simulink model "GS_model"  (R2018b)
settings: Solver=ode5  StartTime=0.0  StopTime=SimuStopTime  FixedStep=T_Simu  RelTol=1e-3
InitFcn:
  | Initial
undefined symbols (not defined in the file or in its folder): Aba10, Aba20, aeroCIP2006_S, aeroCIP2006_X, aeroCIP2006_Y, Agl0, Ass_kS, Ass_n1, Ass_n2, Ass_n3, Ass_n4, Ass_Noise, Ass_R, Ass_Resolution, Ass_TmOrder, AssA_Fix_Abs, AssB_Fix_Abs, AssC_Fix_Abs, AssD_Fix_Abs, AssE_Fix_Aps, AssF_Fix_Aps, C, c_max, c_min, Cd, CenterOfFigNX, CenterOfFigNY, CenterOfFigNZ, CenterOfFigP1, CenterOfFigP2, CenterOfFigPX, CenterOfFigPY, CenterOfFigPZ, Cmu, Crou, DEG2RAD, DiscIntNeverNeededParam, Eg_Dir, Eg_F, Eg_PrepareTime, Eg_r_L_L, Fw_Abf, Fw_Hmax, Fw_J, Fw_Spd0, Fw_Tmax, git_hash_BaseLine, git_hash_Project, Gnss_Noise_Pos, Gnss_Noise_Vel, Gnss_PropgationTime, GyroA_Fix_Abg, GyroA_Noise, GyroB_Fix_Abg, GyroB_Noise, GyroC_Fix_Abg, GyroC_Noise, GyroD_Fix_Abg, GyroD_Noise, h ... (+94)
libraries: simulink x308, sharedutil x46, aerolibutil x37, sharedtransform x31, vrlib x14, aerolibgravity2 x2
(part 1 of 20)
settings Model: PauseTimes=110  ExtModeArmWhenConnect=off  Creator=Think  LastModifiedBy=xiahesong
settings DataIOCC: LimitDataPoints=on  SaveFormat=Array  SaveOutput=off  SaveTime=off  SignalLoggingName=sigsOut
settings DebuggingCC: ReadBeforeWriteMsg=DisableAll  WriteAfterWriteMsg=DisableAll  WriteAfterReadMsg=DisableAll  SaveWithParameterizedLinksMsg=none  MergeDetectMultiDrivingBlocksExec=none  SignalResolutionControl=None  InheritedTsInSrcMsg=none  MultiTaskDSMMsg=none  IntegerOverflowMsg=none  ParameterPrecisionLossMsg=none  ParameterTunabilityLossMsg=none  RootOutportRequireBusObject=error  AllowSymbolicDim=off  StrictBusMsg=ErrorOnBusTreatedAsVector  SFUnexpectedBacktrackingDiag=warning  SFNoUnconditionalDefaultTransitionDiag=warning  IntegerSaturationMsg=none
settings HardwareCC: ProdBitPerPointer=32  ProdBitPerSizeT=32  ProdBitPerPtrDiffT=32  ProdLargestAtomicFloat=None  ProdWordSize=32  ProdHWDeviceType=Intel->x86/Pentium
settings ModelReferenceCC: UpdateModelReferenceTargets=IfOutOfDate  PropagateSignalLabelsOutOfModel=off
settings SFSimCC: SFSimEcho=off  SimUseLocalCustomCode=off
settings RTWCC: SystemTargetFile=NIVeriStand.tlc  TemplateMakefile=NIVeriStand_vc.tmf  Description=DEPRECATED: NI VeriStand Pharlap Real-Time Targets (MATLAB R2018b or earlier)  RTWUseLocalCustomCode=off  RTWCompilerOptimization=on
settings CodeAppCC: StateflowObjectComments=on
settings STFCustomTargetCC: MatFileLogging=on  GRTInterface=on  SystemTargetFile=NIVeriStand.tlc
settings GRTTargetCC: TargetLangStandard=C89/C90 (ANSI)  ParMdlRefBuildCompliant=off  CompOptLevelCompliant=off  ConcurrentExecutionCompliant=off  CombineOutputUpdateFcns=off  CPPClassGenCompliant=off  GRTInterface=on  UseToolchainInfoCompliant=off
settings ConfigComp: CovMetricSettings=dw  CovHtmlReporting=on  CovSaveCumulativeToWorkspaceVar=on  CovSaveSingleToWorkspaceVar=on  CovExternalEMLEnable=off  CovSFcnEnable=off

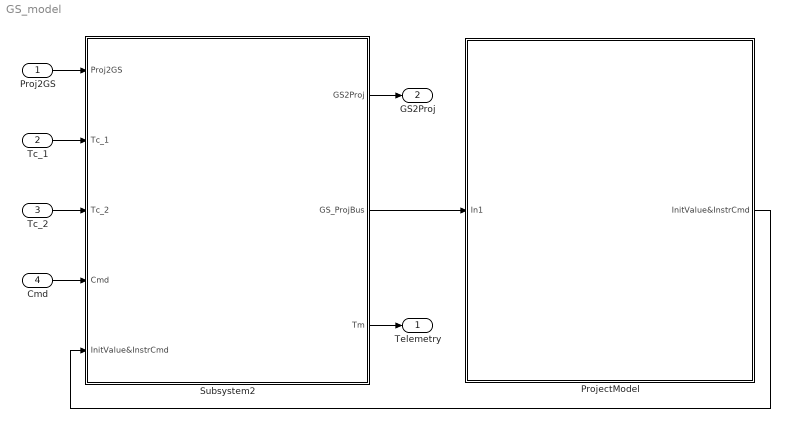
== system GS_model ==
  Proj2GS : Inport
  Tc_1 : Inport  Port=2
  Tc_2 : Inport  Port=3
  Cmd : Inport  Port=4
  ProjectModel : Subsystem
      mask Display: disp('Project Model')
  Subsystem2 : Subsystem
      mask Display: disp('GS_model');
  Telemetry : Outport
  GS2Proj : Outport  Port=2  PortDimensions=166
  wires:
  Tc_1/1 -> Subsystem2/2(Tc_1)
  Tc_2/1 -> Subsystem2/3(Tc_2)
  Cmd/1 -> Subsystem2/4(Cmd)
  Subsystem2/3(Tm) -> Telemetry/1
  Proj2GS/1 -> Subsystem2/1(Proj2GS)
  Subsystem2/1(GS2Proj) -> GS2Proj/1
  ProjectModel/1(InitValue&InstrCmd) -> Subsystem2/5(InitValue&InstrCmd)
  Subsystem2/2(GS_ProjBus) -> ProjectModel/1(In1)

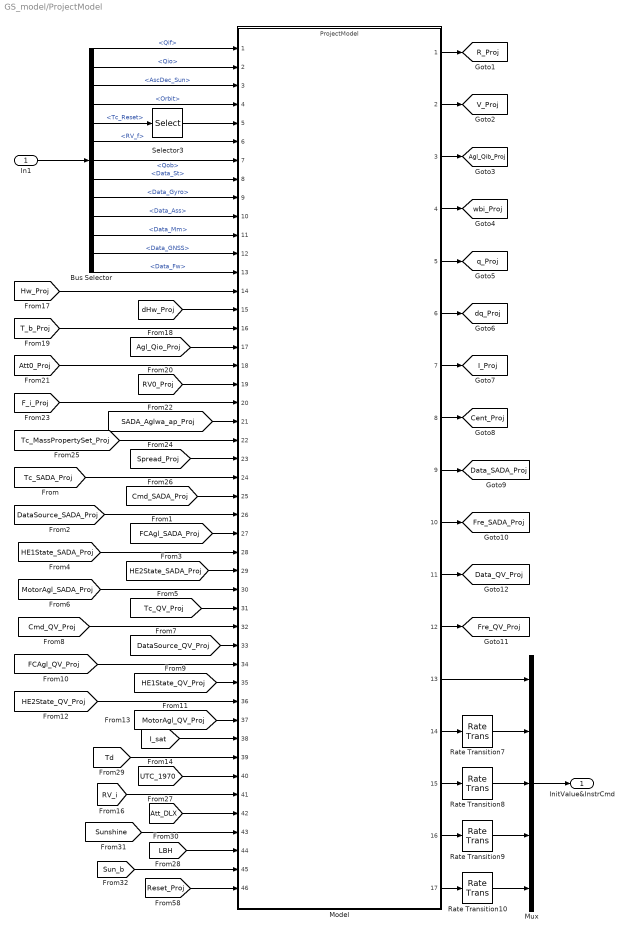
== system GS_model/ProjectModel ==
  In1 : Inport
  Bus Selector : BusSelector  OutputSignals=Qif,Qio,AscDec_Sun,Orbit,Tc_Reset,RV_f,Qob,Data_St,Data_Gyro,Data_Ass,Data_Mm,Data_GNSS,Data_Fw
  Model : ModelReference  ModelNameDialog=ProjectModel  SimulationMode=Normal  ModelReferenceVersion=1.5009
  Mux : Mux  Inputs=5
  Rate Transition{7..10} (4 alike) : RateTransition  OutPortSampleTime=T_Simu
  Selector3 : Selector  InputPortWidth=2  IndexOptions=Index vector (dialog)  Indices=2  OutputSizes=1
  InitValue&InstrCmd : Outport
  tag scope: Agl_Qib_Proj=global, Cent_Proj=global, Data_QV_Proj=global, Data_SADA_Proj=global, Fre_QV_Proj=global, Fre_SADA_Proj=global, I_Proj=global, R_Proj=global, V_Proj=global, dq_Proj=global, q_Proj=global, wbi_Proj=global
  wires:
  Rate Transition8/1 -> Mux/3
  Rate Transition10/1 -> Mux/5
  Rate Transition7/1 -> Mux/2
  Rate Transition9/1 -> Mux/4
  Mux/1 -> InitValue&InstrCmd/1
  Model/1 -> [R_Proj]
  Model/2 -> [V_Proj]
  Model/3 -> [Agl_Qib_Proj]
  Model/4 -> [wbi_Proj]
  Model/5 -> [q_Proj]
  Model/6 -> [dq_Proj]
  Model/7 -> [I_Proj]
  Model/8 -> [Cent_Proj]
  Model/9 -> [Data_SADA_Proj]
  Model/10 -> [Fre_SADA_Proj]
  Model/11 -> [Data_QV_Proj]
  Model/12 -> [Fre_QV_Proj]
  Model/15 -> Rate Transition8/1
  Model/14 -> Rate Transition7/1
  Model/17 -> Rate Transition10/1
  Model/16 -> Rate Transition9/1
  Model/13 -> Mux/1
  In1/1 -> Bus Selector/1
  [HE1State_QV_Proj] -> Model/35
  [MotorAgl_QV_Proj] -> Model/37
  [SADA_Aglwa_ap_Proj] -> Model/21
  [FCAgl_QV_Proj] -> Model/34
  [DataSource_QV_Proj] -> Model/33
  [MotorAgl_SADA_Proj] -> Model/30
  [Tc_QV_Proj] -> Model/31
  [T_b_Proj] -> Model/16
  [FCAgl_SADA_Proj] -> Model/27
  [Spread_Proj] -> Model/23
  [Cmd_SADA_Proj] -> Model/25
  [HE2State_QV_Proj] -> Model/36
  [Agl_Qio_Proj] -> Model/17
  [Tc_SADA_Proj] -> Model/24
  [RV_i] -> Model/41
  [F_i_Proj] -> Model/20
  [Cmd_QV_Proj] -> Model/32
  [dHw_Proj] -> Model/15
  [UTC_1970] -> Model/40
  [HE1State_SADA_Proj] -> Model/28
  [I_sat] -> Model/38
  [HE2State_SADA_Proj] -> Model/29
  [Att0_Proj] -> Model/18
  [RV0_Proj] -> Model/19
  [DataSource_SADA_Proj] -> Model/26
  [Tc_MassPropertySet_Proj] -> Model/22
  [Td] -> Model/39
  [Hw_Proj] -> Model/14
  [Sunshine] -> Model/43
  [Att_DLX] -> Model/42
  [LBH] -> Model/44
  [Sun_b] -> Model/45
  [Reset_Proj] -> Model/46
  Bus Selector/1 -> Model/1  "<Qif>"
  Bus Selector/2 -> Model/2  "<Qio>"
  Bus Selector/3 -> Model/3  "<AscDec_Sun>"
  Bus Selector/4 -> Model/4  "<Orbit>"
  Bus Selector/5 -> Selector3/1  "<Tc_Reset>"
  Bus Selector/6 -> Model/6  "<RV_f>"
  Bus Selector/7 -> Model/7  "<Qob>"
  Bus Selector/8 -> Model/8  "<Data_St>"
  Bus Selector/9 -> Model/9  "<Data_Gyro>"
  Bus Selector/10 -> Model/10  "<Data_Ass>"
  Bus Selector/11 -> Model/11  "<Data_Mm>"
  Bus Selector/12 -> Model/12  "<Data_GNSS>"
  Bus Selector/13 -> Model/13  "<Data_Fw>"
  Selector3/1 -> Model/5

== system GS_model/Subsystem2 ==
  Proj2GS : Inport
  Tc_1 : Inport  Port=2
  Tc_2 : Inport  Port=3
  Cmd : Inport  Port=4
  InitValue&InstrCmd : Inport  Port=5
  " " : Subsystem
      mask Display: disp('Telemetry')
  Bus Creator : BusCreator  Inputs=13
  EquipmentCmd : Subsystem
      mask Display: disp(['Instrument','\n','\n','Cmd'])
  Subsystem : Subsystem
      mask Display: disp('AOCS Model')
  Subsystem1 : Subsystem
      mask Display: disp('Mapping')
  Tc : Subsystem
      mask Display: disp('TC')
  GS2Proj : Outport  PortDimensions=166
  GS_ProjBus : Outport  Port=2
  Tm : Outport  Port=3
  wires:
  InitValue&InstrCmd/1 -> EquipmentCmd/3(InitValue&InstrCmd), Tc/3(InitValue&InstrCmd)
  Tc_2/1 -> Tc/2(Tc_2)
  Cmd/1 -> EquipmentCmd/2(Cmd)
  Tc_1/1 -> Tc/1(Tc_1)
  " "/1(Tm) -> Tm/1
  Tc/18(Tc_Fw) -> Subsystem/18(Tc_Fw), EquipmentCmd/1(Tc_Fw)
  Proj2GS/1 -> Subsystem1/1(In1)
  Subsystem1/1(Out1) -> GS2Proj/1
  Tc/1(Tc_MassProperty) -> Subsystem/1(Tc_MassPropertySet)
  Tc/2(Tc_Sunshine) -> Subsystem/2(Tc_Sunshine)
  Tc/3(Tc_Reset) -> Subsystem/3(Reset)
  Tc/4(Tc_Time0) -> Subsystem/4(Tc_Time0)
  Tc/5(Tc_Orbit0) -> Subsystem/5(Tc_Orbit0)
  Tc/6(Tc_Att0) -> Subsystem/6(Tc_Att0)
  Tc/7(Tc_RemanMag) -> Subsystem/7(Tc_RemanMag)
  Tc/8(Tc_TdCoff) -> Subsystem/8(Tc_TdCoff)
  Tc/9(Tc_St) -> Subsystem/9(Tc_St)
  Tc/10(Tc_Gyro) -> Subsystem/10(Tc_Gyro)
  Tc/11(Tc_Ass) -> Subsystem/11(Tc_Ass)
  Tc/12(Tc_Mm) -> Subsystem/12(Tc_Mm)
  Tc/13(Tc_GNSS) -> Subsystem/13(Tc_GNSS)
  Tc/14(Tc_Mt) -> Subsystem/14(Tc_Mt)
  Tc/15(Tc_SADA) -> Subsystem/15(Tc_SADA)
  Tc/16(Tc_QV) -> Subsystem/16(Tc_QV)
  Tc/17(Tc_Engine) -> Subsystem/17(Tc_Engine)
  Tc/19(Tc_Spread0) -> Subsystem/19(Tc_Spread0)
  EquipmentCmd/1(Cmd_Spread) -> Subsystem/20(Cmd_Spread)
  EquipmentCmd/2(Cmd_Fw) -> Subsystem/21(Cmd_Fw)
  EquipmentCmd/3(Cmd_Mt) -> Subsystem/22(Cmd_Mt)
  EquipmentCmd/4(Cmd_Motor) -> Subsystem/23(Cmd_Motor)
  EquipmentCmd/5(Cmd_Engine) -> Subsystem/24(Cmd_Engine)
  Subsystem/1(Qif) -> Bus Creator/1  "Qif"
  Subsystem/2(Qio) -> Bus Creator/2  "Qio"
  Subsystem/14(Data_St1) -> " "/1(Data_St)
  Subsystem/15(Data_Gyro1) -> " "/2(Data_Gyro)
  Subsystem/16(Data_Ass1) -> " "/3(Data_Ass)
  Subsystem/17(Data_Mm1) -> " "/4(Data_Mm)
  Subsystem/18(Data_GNSS1) -> " "/5(Data_GNSS)
  Subsystem/19(Data_Fw1) -> " "/6(Data_Fw)
  Subsystem/20(Data_Mt) -> " "/7(Data_Mt)
  Subsystem/21(Data_SADA) -> " "/8(Data_SADA)
  Subsystem/22(Data_QV) -> " "/9(Data_QV)
  Subsystem/3(AscDec_Sun) -> Bus Creator/3  "AscDec_Sun"
  Subsystem/4(Orbit) -> Bus Creator/4  "Orbit"
  Subsystem/5(Tc_Reset) -> Bus Creator/5  "Tc_Reset"
  Subsystem/6(RV_f) -> Bus Creator/6  "RV_f"
  Subsystem/7(Qob) -> Bus Creator/7  "Qob"
  Subsystem/8(Data_St) -> Bus Creator/8  "Data_St"
  Subsystem/9(Data_Gyro) -> Bus Creator/9  "Data_Gyro"
  Subsystem/10(Data_Ass) -> Bus Creator/10  "Data_Ass"
  Subsystem/11(Data_Mm) -> Bus Creator/11  "Data_Mm"
  Subsystem/12(Data_GNSS) -> Bus Creator/12  "Data_GNSS"
  Subsystem/13(Data_Fw) -> Bus Creator/13  "Data_Fw"
  Bus Creator/1 -> GS_ProjBus/1

== system GS_model/Subsystem2/  ==
  Data_St : Inport
  Data_Gyro : Inport  Port=2
  Data_Ass : Inport  Port=3
  Data_Mm : Inport  Port=4
  Data_GNSS : Inport  Port=5
  Data_Fw : Inport  Port=6
  Data_Mt : Inport  Port=7
  Data_SADA : Inport  Port=8
  Data_QV : Inport  Port=9
  DynTelemetry : Subsystem
      mask Display: disp('TM_Dyn')
  Hash : Subsystem
      mask Display: disp('TM_Hash')
  Mux : Mux  Inputs=11
  Reshape : Reshape  OutputDimensionality=Row vector (2-D)
  Subsystem : Subsystem
      mask Display: disp('TM_Ass');
  Subsystem1 : Subsystem
      mask Display: disp('TM_SADA');
  Subsystem2 : Subsystem
      mask Display: disp('TM_QV');
  Tm : Outport  VectorParamsAs1DForOutWhenUnconnected=on
  wires:
  DynTelemetry/1(DynTelemetry) -> Mux/1
  Hash/1(Out1) -> Mux/2
  Data_St/1 -> Mux/3
  Data_Gyro/1 -> Mux/4
  Data_Mm/1 -> Mux/5
  Data_GNSS/1 -> Mux/7
  Data_Fw/1 -> Mux/8
  Data_Mt/1 -> Mux/9
  Data_SADA/1 -> Subsystem1/1(Data_SADA)
  Data_QV/1 -> Subsystem2/1(Data_QV)
  Mux/1 -> Reshape/1
  Data_Ass/1 -> Subsystem/1(Data_Ass)
  Subsystem/1(Out6) -> Mux/6
  Reshape/1 -> Tm/1
  Subsystem1/1(Out6) -> Mux/10
  Subsystem2/1(Out6) -> Mux/11

== system GS_model/Subsystem2/EquipmentCmd ==
  Tc_Fw : Inport
  Cmd : Inport  Port=2
  InitValue&InstrCmd : Inport  Port=3
  Demux : Demux  Outputs=[42;25;40;1;4]
  Engine1 : Subsystem
      mask Display: disp('Cmd_Engine')
  Fw : Subsystem
      mask Display: disp('Cmd_FW')
  Fw1 : Subsystem
      mask Display: disp('Cmd_FW')
  Motor : Subsystem
      mask Display: disp('Cmd_Motor')
  Motor1 : Subsystem
      mask Display: disp('Cmd_Motor')
  Mt : Subsystem
      mask Display: disp('Cmd_Mt')
  Mt1 : Subsystem
      mask Display: disp('Cmd_Mt')
  PanelSpread : Subsystem
      mask Display: disp('PanelSpread')
  Selector : Selector  InputPortWidth=97  IndexOptions=Index vector (dialog)  Indices=44:97  OutputSizes=1
  Selector1 : Selector  InputPortWidth=54  IndexOptions=Index vector (dialog)  Indices=1:18  OutputSizes=1
  Selector2 : Selector  InputPortWidth=54  IndexOptions=Index vector (dialog)  Indices=19:30  OutputSizes=1
  Selector3 : Selector  InputPortWidth=54  IndexOptions=Index vector (dialog)  Indices=31:50  OutputSizes=1
  Selector4 : Selector  InputPortWidth=54  IndexOptions=Index vector (dialog)  Indices=51:54  OutputSizes=1
  Cmd_Spread : Outport
  Cmd_Fw : Outport  Port=2
  Cmd_Mt : Outport  Port=3
  Cmd_Motor : Outport  Port=4
  Cmd_Engine : Outport  Port=5
  wires:
  Fw1/1(Cmd_Fw) -> Cmd_Fw/1
  Mt1/1(Cmd_Mt) -> Cmd_Mt/1
  Motor1/1(Cmd_Moror) -> Cmd_Motor/1
  PanelSpread/1(Cmd_Spread) -> Cmd_Spread/1
  Tc_Fw/1 -> Fw1/1(Tc_Fw)
  Fw/1(Cmd_FwA) -> Fw1/3(in1)
  Fw/2(Cmd_FwB) -> Fw1/4(in2)
  Fw/3(Cmd_FwC) -> Fw1/5(in3)
  Fw/4(Cmd_FwD) -> Fw1/6(in4)
  Fw/5(Cmd_FwE) -> Fw1/7(in5)
  Fw/6(Cmd_FwF) -> Fw1/8(in6)
  Mt/1(Cmd_Mt_UDP) -> Mt1/2(UDP)
  Mt/2(Cmd_Mt_FC) -> Mt1/3(FC)
  Mt/3(Cmd_Mt_DataSour) -> Mt1/4(DataSource)
  Motor/1(Cmd_Moror) -> Motor1/2(Cmd_Motor)
  Motor/2(SadaStep_FC) -> Motor1/3(SadaStep_FC)
  Motor/3(QvAgl_FC) -> Motor1/4(QVAgl_FC)
  Motor/4(DataSource_SADA) -> Motor1/5(DataSource_SADA)
  Demux/5 -> Engine1/2(In1)
  Engine1/1(Cmd_Engine) -> Cmd_Engine/1
  Selector/1 -> [InstrCmd]
  InitValue&InstrCmd/1 -> Selector/1
  Motor/5(DataSource_QV) -> Motor1/6(DataSource_QV)
  Demux/4 -> PanelSpread/1(In1)
  Demux/3 -> Motor/1(In1)
  Demux/2 -> Mt/1(In1)
  Demux/1 -> Fw/1(In1)
  Cmd/1 -> Demux/1
  [InstrCmd] -> Selector1/1
  Selector1/1 -> Fw1/2(Hw_Cmd_Test)
  Selector2/1 -> Mt1/1(M_Cmd_Test)
  [InstrCmd] -> Selector2/1
  Selector3/1 -> Motor1/1(SADAQV_Cmd_Test)
  [InstrCmd] -> Selector3/1
  [InstrCmd] -> Selector4/1
  Selector4/1 -> Engine1/1(Engine_Cmd_Test)

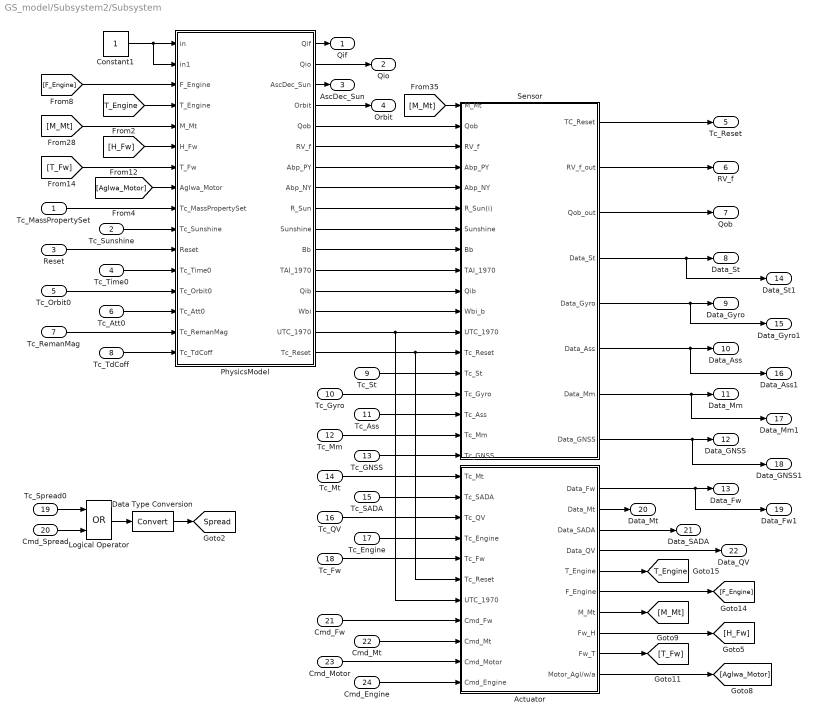
== system GS_model/Subsystem2/Subsystem ==
  Tc_MassPropertySet : Inport
  Tc_Sunshine : Inport  Port=2
  Reset : Inport  Port=3
  Tc_Time0 : Inport  Port=4
  Tc_Orbit0 : Inport  Port=5
  Tc_Att0 : Inport  Port=6
  Tc_RemanMag : Inport  Port=7
  Tc_TdCoff : Inport  Port=8
  Tc_St : Inport  Port=9
  Tc_Gyro : Inport  Port=10
  Tc_Ass : Inport  Port=11
  Tc_Mm : Inport  Port=12
  Tc_GNSS : Inport  Port=13
  Tc_Mt : Inport  Port=14
  Tc_SADA : Inport  Port=15
  Tc_QV : Inport  Port=16
  Tc_Engine : Inport  Port=17
  Tc_Fw : Inport  Port=18
  Tc_Spread0 : Inport  Port=19
  Cmd_Spread : Inport  Port=20
  Cmd_Fw : Inport  Port=21
  Cmd_Mt : Inport  Port=22
  Cmd_Motor : Inport  Port=23
  Cmd_Engine : Inport  Port=24
  Actuator : Subsystem
      mask Display: disp('Actuator');
  Constant1 : Constant
  Data Type Conversion : DataTypeConversion
  Logical Operator : Logic  Operator=OR  AllPortsSameDT=off  OutDataTypeStr=boolean
  PhysicsModel : Subsystem
      mask Display: disp('System')
  Sensor : Subsystem
      mask Display: disp('Sensor');
  Qif : Outport
  Qio : Outport  Port=2
  AscDec_Sun : Outport  Port=3
  Orbit : Outport  Port=4
  Tc_Reset : Outport  Port=5
  RV_f : Outport  Port=6
  Qob : Outport  Port=7
  Data_St : Outport  Port=8
  Data_Gyro : Outport  Port=9
  Data_Ass : Outport  Port=10
  Data_Mm : Outport  Port=11
  Data_GNSS : Outport  Port=12
  Data_Fw : Outport  Port=13
  Data_St1 : Outport  Port=14
  Data_Gyro1 : Outport  Port=15
  Data_Ass1 : Outport  Port=16
  Data_Mm1 : Outport  Port=17
  Data_GNSS1 : Outport  Port=18
  Data_Fw1 : Outport  Port=19
  Data_Mt : Outport  Port=20
  Data_SADA : Outport  Port=21
  Data_QV : Outport  Port=22
  tag scope: Spread=global, T_Engine=global
  wires:
  PhysicsModel/6(RV_f) -> Sensor/3(RV_f)
  PhysicsModel/9(R_Sun) -> Sensor/6(R_Sun(i))
  Actuator/1(Data_Fw) -> Data_Fw1/1, Data_Fw/1
  PhysicsModel/5(Qob) -> Sensor/2(Qob)
  Constant1/1 -> PhysicsModel/2(in1), PhysicsModel/1(in)
  PhysicsModel/7(Abp_PY) -> Sensor/4(Abp_PY)
  Sensor/7(Data_Mm) -> Data_Mm1/1, Data_Mm/1
  Actuator/6(F_Engine) -> [F_Engine]
  PhysicsModel/2(Qio) -> Qio/1
  PhysicsModel/15(UTC_1970) -> Actuator/7(UTC_1970), Sensor/12(UTC_1970)
  Sensor/2(RV_f_out) -> RV_f/1
  Actuator/10(Motor_Agl/w/a) -> [Aglwa_Motor]
  Actuator/7(M_Mt) -> [M_Mt]
  Actuator/8(Fw_H) -> [H_Fw]
  Actuator/3(Data_SADA) -> Data_SADA/1
  Actuator/4(Data_QV) -> Data_QV/1
  [H_Fw] -> PhysicsModel/6(H_Fw)
  Logical Operator/1 -> Data Type Conversion/1
  PhysicsModel/12(TAI_1970) -> Sensor/9(TAI_1970)
  Sensor/8(Data_GNSS) -> Data_GNSS1/1, Data_GNSS/1
  PhysicsModel/13(Qib) -> Sensor/10(Qib)
  Sensor/5(Data_Gyro) -> Data_Gyro1/1, Data_Gyro/1
  PhysicsModel/4("Orbit ") -> Orbit/1
  PhysicsModel/3(AscDec_Sun) -> AscDec_Sun/1
  Actuator/2(Data_Mt) -> Data_Mt/1
  [T_Engine] -> PhysicsModel/4(T_Engine)
  [F_Engine] -> PhysicsModel/3(F_Engine)
  Data Type Conversion/1 -> [Spread]
  Actuator/5(T_Engine) -> [T_Engine]
  [M_Mt] -> PhysicsModel/5(M_Mt)
  [T_Fw] -> PhysicsModel/7(T_Fw)
  Sensor/6(Data_Ass) -> Data_Ass1/1, Data_Ass/1
  PhysicsModel/1(Qif) -> Qif/1
  [M_Mt] -> Sensor/1(M_Mt)
  Actuator/9(Fw_T) -> [T_Fw]
  PhysicsModel/10(Sunshine) -> Sensor/7(Sunshine)
  PhysicsModel/14(Wbi) -> Sensor/11(Wbi_b)
  Sensor/4(Data_St) -> Data_St1/1, Data_St/1
  PhysicsModel/16(Tc_Reset) -> Actuator/6(Tc_Reset), Sensor/13(Tc_Reset)
  [Aglwa_Motor] -> PhysicsModel/8(Aglwa_Motor)
  PhysicsModel/8(Abp_NY) -> Sensor/5(Abp_NY)
  Sensor/1(TC_Reset) -> Tc_Reset/1
  PhysicsModel/11(Bb) -> Sensor/8(Bb)
  Sensor/3(Qob_out) -> Qob/1
  Tc_MassPropertySet/1 -> PhysicsModel/9(Tc_MassPropertySet)
  Tc_Orbit0/1 -> PhysicsModel/13(Tc_Orbit0)
  Tc_RemanMag/1 -> PhysicsModel/15(Tc_RemanMag)
  Reset/1 -> PhysicsModel/11(Reset)
  Tc_Att0/1 -> PhysicsModel/14(Tc_Att0)
  Tc_TdCoff/1 -> PhysicsModel/16(Tc_TdCoff)
  Tc_Sunshine/1 -> PhysicsModel/10(Tc_Sunshine)
  Tc_Time0/1 -> PhysicsModel/12(Tc_Time0)
  Tc_SADA/1 -> Actuator/2(Tc_SADA)
  Tc_Mt/1 -> Actuator/1(Tc_Mt)
  Tc_Engine/1 -> Actuator/4(Tc_Engine)
  Tc_St/1 -> Sensor/14(Tc_St)
  Tc_GNSS/1 -> Sensor/18(Tc_GNSS)
  Tc_Mm/1 -> Sensor/17(Tc_Mm)
  Tc_Ass/1 -> Sensor/16(Tc_Ass)
  Tc_Gyro/1 -> Sensor/15(Tc_Gyro)
  Tc_Fw/1 -> Actuator/5(Tc_Fw)
  Tc_QV/1 -> Actuator/3(Tc_QV)
  Tc_Spread0/1 -> Logical Operator/1
  Cmd_Spread/1 -> Logical Operator/2
  Cmd_Fw/1 -> Actuator/8(Cmd_Fw)
  Cmd_Mt/1 -> Actuator/9(Cmd_Mt)
  Cmd_Engine/1 -> Actuator/11(Cmd_Engine)
  Cmd_Motor/1 -> Actuator/10(Cmd_Motor)

== system GS_model/Subsystem2/Subsystem1 ==
  In1 : Inport
  Demux : Demux  Outputs=[3;3;3;3;10;10;9;3;186;6;124;4]
  Mux1 : Mux  Inputs=[1;3;3;3;3;6;6;3;30;4;8;17;12;6;6;6;6;6;9;8;4;4;4;4;4]
  Out1 : Outport
  tag scope: Agl_Qib_Test=global, Cent_Test=global, Data_QV_Test=global, Data_SADA_Test=global, Fre_QV_Test=global, Fre_SADA_Test=global, I_Test=global, R_Test=global, V_Test=global, dq_Test=global, q_Test=global, wbi_Test=global
  wires:
  Demux/12 -> [Fre_QV_Test]
  Demux/4 -> [wbi_Test]
  Demux/1 -> [R_Test]
  Demux/3 -> [Agl_Qib_Test]
  Demux/7 -> [I_Test]
  Demux/5 -> [q_Test]
  Demux/6 -> [dq_Test]
  Demux/2 -> [V_Test]
  Demux/8 -> [Cent_Test]
  In1/1 -> Demux/1
  Mux1/1 -> Out1/1
  [HE2State_QV_Proj] -> Mux1/24
  [HE1State_SADA_Proj] -> Mux1/16
  [Reset_Proj] -> Mux1/1
  [Tc_SADA_Proj] -> Mux1/12
  [Tc_QV_Proj] -> Mux1/19
  [Att0_Proj] -> Mux1/6
  [Cmd_QV_Proj] -> Mux1/20
  [FCAgl_QV_Proj] -> Mux1/22
  [RV0_Proj] -> Mux1/7
  [Tc_MassPropertySet_Proj] -> Mux1/10
  [dHw_Proj] -> Mux1/3
  [FCAgl_SADA_Proj] -> Mux1/15
  [MotorAgl_QV_Proj] -> Mux1/25
  [T_b_Proj] -> Mux1/4
  [Agl_Qio_Proj] -> Mux1/5
  [HE2State_SADA_Proj] -> Mux1/17
  [SADA_Aglwa_ap_Proj] -> Mux1/9
  [DataSource_SADA_Proj] -> Mux1/14
  [DataSource_QV_Proj] -> Mux1/21
  [F_i_Proj] -> Mux1/8
  [Hw_Proj] -> Mux1/2
  [HE1State_QV_Proj] -> Mux1/23
  [Spread_Proj] -> Mux1/11
  [MotorAgl_SADA_Proj] -> Mux1/18
  [Cmd_SADA_Proj] -> Mux1/13
  Demux/9 -> [Data_SADA_Test]
  Demux/10 -> [Fre_SADA_Test]
  Demux/11 -> [Data_QV_Test]

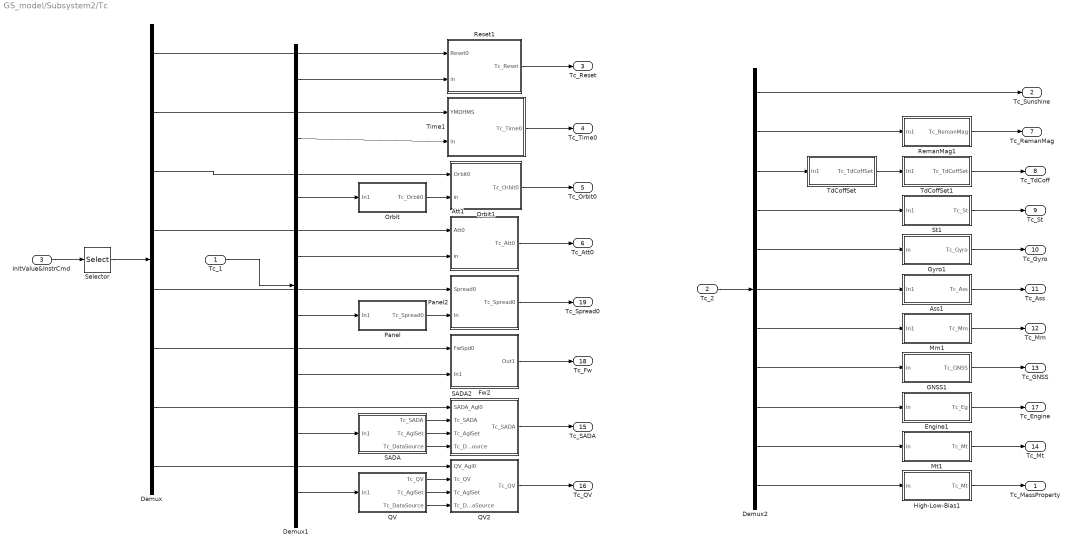
== system GS_model/Subsystem2/Tc ==
  Tc_1 : Inport
  Tc_2 : Inport  Port=2
  InitValue&InstrCmd : Inport  Port=3
  Ass1 : Subsystem
  Att1 : Subsystem
  Demux : Demux  Outputs=[1;6;6;6;8;6;6;4]
  Demux1 : Demux  Outputs=[1;1;6;6;2;17;24;14]
  Demux2 : Demux  Outputs=[2;3;3;26;24;17;20;16;11;9;4]
  Engine1 : Subsystem
  Fw2 : Subsystem
  GNSS1 : Subsystem
  Gyro1 : Subsystem
  High-Low-Bias1 : Subsystem
  Mm1 : Subsystem
  Mt1 : Subsystem
  Orbit : Subsystem
  Orbit1 : Subsystem
  Panel : Subsystem
  Panel2 : Subsystem
  QV : Subsystem
  QV2 : Subsystem
  RemanMag1 : Subsystem
  Reset1 : Subsystem
  SADA : Subsystem
  SADA2 : Subsystem
  Selector : Selector  InputPortWidth=97  IndexOptions=Index vector (dialog)  Indices=1:43  OutputSizes=1
  St1 : Subsystem
  TdCoffSet : Subsystem
  TdCoffSet1 : Subsystem
  Time1 : Subsystem
  Tc_MassProperty : Outport
  Tc_Sunshine : Outport  Port=2
  Tc_Reset : Outport  Port=3
  Tc_Time0 : Outport  Port=4
  Tc_Orbit0 : Outport  Port=5
  Tc_Att0 : Outport  Port=6
  Tc_RemanMag : Outport  Port=7
  Tc_TdCoff : Outport  Port=8
  Tc_St : Outport  Port=9
  Tc_Gyro : Outport  Port=10
  Tc_Ass : Outport  Port=11
  Tc_Mm : Outport  Port=12
  Tc_GNSS : Outport  Port=13
  Tc_Mt : Outport  Port=14
  Tc_SADA : Outport  Port=15
  Tc_QV : Outport  Port=16
  Tc_Engine : Outport  Port=17
  Tc_Fw : Outport  Port=18
  Tc_Spread0 : Outport  Port=19
  wires:
  St1/1(Tc_St) -> Tc_St/1
  Gyro1/1(Tc_Gyro) -> Tc_Gyro/1
  Orbit1/1(Tc_Orbit0) -> Tc_Orbit0/1
  Att1/1(Tc_Att0) -> Tc_Att0/1
  Ass1/1(Tc_Ass) -> Tc_Ass/1
  Mm1/1(Tc_Mm) -> Tc_Mm/1
  Mt1/1(Tc_Mt) -> Tc_Mt/1
  Fw2/1(Out1) -> Tc_Fw/1
  SADA2/1(Tc_SADA) -> Tc_SADA/1
  QV2/1(Tc_QV) -> Tc_QV/1
  RemanMag1/1(Tc_RemanMag) -> Tc_RemanMag/1
  Time1/1(Tc_Time0) -> Tc_Time0/1
  GNSS1/1(Tc_GNSS) -> Tc_GNSS/1
  Reset1/1("Tc_Reset ") -> Tc_Reset/1
  TdCoffSet1/1(Tc_TdCoffSet) -> Tc_TdCoff/1
  Panel2/1(Tc_Spread0) -> Tc_Spread0/1
  InitValue&InstrCmd/1 -> Selector/1
  Demux/1 -> Reset1/1(Reset0)
  Demux/2 -> Time1/1(YMDHMS)
  Demux/3 -> Orbit1/1(Orbit0)
  Demux/4 -> Att1/1(Att0)
  Demux/5 -> Panel2/1(Spread0)
  Demux/6 -> Fw2/1(FwSpd0)
  Demux/7 -> SADA2/1(SADA_Agl0)
  Demux/8 -> QV2/1(QV_Agl0)
  Demux1/1 -> Reset1/2(in)
  Demux1/2 -> Time1/2(in)
  Orbit/1(Tc_Orbit0) -> Orbit1/2(in)
  Demux1/4 -> Att1/2(in)
  Panel/1(Tc_Spread0) -> Panel2/2(In)
  Demux1/6 -> Fw2/2(In1)
  SADA/1(Tc_SADA) -> SADA2/2("Tc_SADA ")
  SADA/2(Tc_AglSet) -> SADA2/3(Tc_AglSet)
  QV/1(Tc_QV) -> QV2/2("Tc_QV ")
  QV/2(Tc_AglSet) -> QV2/3(Tc_AglSet)
  Demux2/2 -> RemanMag1/1(In1)
  TdCoffSet/1(Tc_TdCoffSet) -> TdCoffSet1/1(In1)
  Demux2/4 -> St1/1(In1)
  Demux2/5 -> Gyro1/1(in)
  Demux2/6 -> Ass1/1(In1)
  Demux2/7 -> Mm1/1(In1)
  Demux2/10 -> Mt1/1(in)
  Demux2/1 -> Tc_Sunshine/1
  Demux2/11 -> High-Low-Bias1/1(in)
  High-Low-Bias1/1(Tc_Mt) -> Tc_MassProperty/1
  Demux2/9 -> Engine1/1(in)
  Engine1/1(Tc_Eg) -> Tc_Engine/1
  SADA/3(Tc_DataSource) -> SADA2/4(Tc_DataSource)
  Selector/1 -> Demux/1
  Demux2/8 -> GNSS1/1(in)
  Tc_1/1 -> Demux1/1
  Demux1/8 -> QV/1(In1)
  Demux1/7 -> SADA/1(In1)
  Demux1/5 -> Panel/1(In1)
  Demux1/3 -> Orbit/1(In1)
  QV/3(Tc_DataSource) -> QV2/4(Tc_DataSource)
  Demux2/3 -> TdCoffSet/1(In1)
  Tc_2/1 -> Demux2/1

== system GS_model/Subsystem2/ /DynTelemetry ==
  Add3 : Sum  Inputs=-+
  Constant1 : Constant  Value=[0;0;0]
  Constant2 : Constant  Value=[0;0]
  Constant3 : Constant  Value=[0;0;0;0;0]
  Fcn : Fcn  Expr=u(1)+u(2)*2^1+u(3)*2^2+u(4)*2^3+u(5)*2^4+u(6)*2^5+u(7)*2^6+u(8)*2^7
  Gain{,2..4} (4 alike) : Gain  Gain=RAD2DEG
  Gain1 : Gain  Gain=1e06  SaturateOnIntegerOverflow=on  OutDataTypeStr=Inherit: Same as input  ParamDataTypeStr=Inherit: Same as input
  Mux : Mux  Inputs=27
  Rounding Function1 : Rounding
  Rounding Function2 : Rounding
  Selector6 : Selector  InputPortWidth=10  IndexOptions=Index vector (dialog)  Indices=[1 2 3]  OutputSizes=1
  Selector7 : Selector  InputPortWidth=10  IndexOptions=Index vector (dialog)  Indices=[6 7 8]  OutputSizes=1
  Subsystem : Subsystem
  TM_Orbit : Subsystem
  DynTelemetry : Outport  VectorParamsAs1DForOutWhenUnconnected=on
  wires:
  Gain1/1 -> Rounding Function2/1
  Add3/1 -> Gain1/1
  [UTC_1970] -> Add3/2, Rounding Function1/1
  Rounding Function1/1 -> Add3/1, Mux/1
  [Spread] -> Fcn/1
  [q_panel] -> Selector7/1, Selector6/1
  Rounding Function2/1 -> Mux/2
  [RV_i] -> Mux/3
  [DisTg] -> Mux/4
  [DisTs] -> Mux/5
  [DisTm] -> Mux/6
  [T_Engine] -> Mux/7
  [DisTa] -> Mux/8
  [T_Fw3] -> Mux/9
  [Tm] -> Mux/10
  [Wbi] -> Gain2/1
  [Wbo] -> Gain/1
  Constant1/1 -> Mux/13
  [Qib] -> Mux/14
  [Euler_o] -> Gain3/1
  [Euler_i] -> Gain4/1
  TM_Orbit/1(Out1) -> Mux/17
  Constant3/1 -> Mux/18
  [Sun_b] -> Mux/19
  [TM_SADA_Agl] -> Mux/20
  [Sunshine] -> Mux/21
  Fcn/1 -> Mux/22
  [Agl_StSunEarth] -> Mux/23
  Constant2/1 -> Mux/24
  Subsystem/1(Out1) -> Mux/25
  Selector6/1 -> Mux/26
  Selector7/1 -> Mux/27
  Mux/1 -> DynTelemetry/1
  Gain/1 -> Mux/12
  Gain2/1 -> Mux/11
  Gain3/1 -> Mux/15
  Gain4/1 -> Mux/16

== system GS_model/Subsystem2/ /Hash ==
  Constant : Constant  Value=SatID
  Constant1 : Constant  Value=git_hash_Project
  Constant2 : Constant  Value=git_hash_BaseLine
  Mux : Mux  Inputs=3
  Out1 : Outport  VectorParamsAs1DForOutWhenUnconnected=on
  wires:
  Constant/1 -> Mux/1
  Constant1/1 -> Mux/2
  Constant2/1 -> Mux/3
  Mux/1 -> Out1/1

== system GS_model/Subsystem2/ /Subsystem ==
  Data_Ass : Inport
  Constant : Constant  Value=Ass_TmOrder
  Demux : Demux  Outputs=6
  MATLAB Function : MATLAB Function  TreatAsAtomicUnit=on
  Out6 : Outport  VectorParamsAs1DForOutWhenUnconnected=on
  wires:
  MATLAB Function/1(Ass_Tm) -> Out6/1
  Constant/1 -> MATLAB Function/7(Ass_TmOrder)
  Demux/1 -> MATLAB Function/1(AssA)
  Demux/2 -> MATLAB Function/2(AssB)
  Demux/3 -> MATLAB Function/3(AssC)
  Demux/4 -> MATLAB Function/4(AssD)
  Demux/5 -> MATLAB Function/5(AssE)
  Demux/6 -> MATLAB Function/6(AssF)
  Data_Ass/1 -> Demux/1

== system GS_model/Subsystem2/ /Subsystem1 ==
  Data_SADA : Inport
  Demux : Demux  Outputs=[1;1;186]
  Mux : Mux  Inputs=6
  Mux1 : Mux  Inputs=6
  Mux2 : Mux  Inputs=3
  Out6 : Outport  VectorParamsAs1DForOutWhenUnconnected=on
  wires:
  Data_SADA/1 -> Demux/1
  Mux2/1 -> Out6/1
  Demux/1 -> Mux/2, Mux/1, Mux/3, Mux/4, Mux/6, Mux/5
  Demux/2 -> Mux1/1, Mux1/2, Mux1/3, Mux1/6, Mux1/5, Mux1/4
  Demux/3 -> Mux2/3
  Mux1/1 -> Mux2/2
  Mux/1 -> Mux2/1

== system GS_model/Subsystem2/ /Subsystem2 ==
  Data_QV : Inport
  Demux : Demux  Outputs=[1;1;124]
  Mux : Mux
  Mux1 : Mux
  Mux2 : Mux  Inputs=3
  Out6 : Outport  VectorParamsAs1DForOutWhenUnconnected=on
  wires:
  Mux/1 -> Mux2/1
  Mux1/1 -> Mux2/2
  Demux/3 -> Mux2/3
  Demux/2 -> Mux1/1, Mux1/2, Mux1/4, Mux1/3
  Demux/1 -> Mux/1, Mux/2, Mux/3, Mux/4
  Mux2/1 -> Out6/1
  Data_QV/1 -> Demux/1

== system GS_model/Subsystem2/EquipmentCmd/Engine1 ==
  Engine_Cmd_Test : Inport
  In1 : Inport  Port=2
  Constant2 : Constant  Value=TestMode
  Switch : Switch  Criteria=u2 > Threshold  Threshold=0.5
  Cmd_Engine : Outport
  wires:
  In1/1 -> Switch/3
  Engine_Cmd_Test/1 -> Switch/1
  Switch/1 -> Cmd_Engine/1
  Constant2/1 -> Switch/2

== system GS_model/Subsystem2/EquipmentCmd/Fw ==
  In1 : Inport
  Demux : Demux  Outputs=6
  Subsystem : Subsystem
  Subsystem1 : Subsystem
  Subsystem2 : Subsystem
  Subsystem3 : Subsystem
  Subsystem4 : Subsystem
  Subsystem5 : Subsystem
  Cmd_FwA : Outport
  Cmd_FwB : Outport  Port=2
  Cmd_FwC : Outport  Port=3
  Cmd_FwD : Outport  Port=4
  Cmd_FwE : Outport  Port=5
  Cmd_FwF : Outport  Port=6
  wires:
  Subsystem5/1(Cmd_FW) -> Cmd_FwF/1
  Subsystem4/1(Cmd_FW) -> Cmd_FwE/1
  Subsystem3/1(Cmd_FW) -> Cmd_FwD/1
  Subsystem2/1(Cmd_FW) -> Cmd_FwC/1
  Subsystem1/1(Cmd_FW) -> Cmd_FwB/1
  Subsystem/1(Cmd_FW) -> Cmd_FwA/1
  Demux/1 -> Subsystem/1(In1)
  Demux/2 -> Subsystem1/1(In1)
  Demux/3 -> Subsystem2/1(In1)
  Demux/4 -> Subsystem3/1(In1)
  Demux/5 -> Subsystem4/1(In1)
  Demux/6 -> Subsystem5/1(In1)
  In1/1 -> Demux/1

== system GS_model/Subsystem2/EquipmentCmd/Fw1 ==
  note: FwA Mode/Spd/T
      | FwB Mode/Spd/T
      | ...
      | FwF Mode/Spd/T
  Tc_Fw : Inport
  Hw_Cmd_Test : Inport  Port=2
  in1 : Inport  Port=3
  in2 : Inport  Port=4
  in3 : Inport  Port=5
  in4 : Inport  Port=6
  in5 : Inport  Port=7
  in6 : Inport  Port=8
  Constant4 : Constant  Value=TestMode
  Data Store Memory1 : DataStoreMemory  DataStoreName=Cmd_FwB  ReadBeforeWriteMsg=warning  WriteAfterWriteMsg=warning  WriteAfterReadMsg=warning  InitialValue=zeros(10,1)  ShowAdditionalParam=off
  Data Store Memory2 : DataStoreMemory  DataStoreName=Cmd_FwC  ReadBeforeWriteMsg=warning  WriteAfterWriteMsg=warning  WriteAfterReadMsg=warning  InitialValue=zeros(10,1)  ShowAdditionalParam=off
  Data Store Memory3 : DataStoreMemory  DataStoreName=Cmd_FwD  ReadBeforeWriteMsg=warning  WriteAfterWriteMsg=warning  WriteAfterReadMsg=warning  InitialValue=zeros(10,1)  ShowAdditionalParam=off
  Data Store Memory4 : DataStoreMemory  DataStoreName=Cmd_FwA  ReadBeforeWriteMsg=warning  WriteAfterWriteMsg=warning  WriteAfterReadMsg=warning  InitialValue=zeros(10,1)  ShowAdditionalParam=off
  Data Store Memory5 : DataStoreMemory  DataStoreName=Cmd_FwE  ReadBeforeWriteMsg=warning  WriteAfterWriteMsg=warning  WriteAfterReadMsg=warning  InitialValue=zeros(10,1)  ShowAdditionalParam=off
  Data Store Memory6 : DataStoreMemory  DataStoreName=Cmd_FwF  ReadBeforeWriteMsg=warning  WriteAfterWriteMsg=warning  WriteAfterReadMsg=warning  InitialValue=zeros(10,1)  ShowAdditionalParam=off
  Data Store Read1 : DataStoreRead  DataStoreName=Cmd_FwB
  Data Store Read2 : DataStoreRead  DataStoreName=Cmd_FwC
  Data Store Read3 : DataStoreRead  DataStoreName=Cmd_FwD
  Data Store Read4 : DataStoreRead  DataStoreName=Cmd_FwA
  Data Store Read5 : DataStoreRead  DataStoreName=Cmd_FwE
  Data Store Read6 : DataStoreRead  DataStoreName=Cmd_FwF
  Data Store Write1 : DataStoreWrite  DataStoreName=Cmd_FwB
  Data Store Write2 : DataStoreWrite  DataStoreName=Cmd_FwC
  Data Store Write3 : DataStoreWrite  DataStoreName=Cmd_FwD
  Data Store Write4 : DataStoreWrite  DataStoreName=Cmd_FwA
  Data Store Write5 : DataStoreWrite  DataStoreName=Cmd_FwE
  Data Store Write6 : DataStoreWrite  DataStoreName=Cmd_FwF
  Subsystem7 : Subsystem
  Switch1 : Switch  Criteria=u2 > Threshold  Threshold=0.5
  Cmd_Fw : Outport
  wires:
  Switch1/1 -> Cmd_Fw/1
  Data Store Read4/1 -> Subsystem7/2(FwA_Cmd)
  Data Store Read1/1 -> Subsystem7/3(FwB_Cmd)
  Data Store Read2/1 -> Subsystem7/4(FwC_Cmd)
  Data Store Read3/1 -> Subsystem7/5(FwD_Cmd)
  Data Store Read5/1 -> Subsystem7/6(FwE_Cmd)
  Data Store Read6/1 -> Subsystem7/7(FwF_Cmd)
  Constant4/1 -> Switch1/2
  Tc_Fw/1 -> Subsystem7/1(Tc_Fw)
  Subsystem7/1(Fw_Mode/Spd/T) -> Switch1/3
  Hw_Cmd_Test/1 -> Switch1/1
  in1/1 -> Data Store Write4/1
  in2/1 -> Data Store Write1/1
  in3/1 -> Data Store Write2/1
  in4/1 -> Data Store Write3/1
  in5/1 -> Data Store Write5/1
  in6/1 -> Data Store Write6/1

== system GS_model/Subsystem2/EquipmentCmd/Motor ==
  In1 : Inport
  Demux : Demux  Outputs=[20;6;4;6;4]
  Cmd_Moror : Outport
  SadaStep_FC : Outport  Port=2
  QvAgl_FC : Outport  Port=3
  DataSource_SADA : Outport  Port=4
  DataSource_QV : Outport  Port=5
  wires:
  Demux/4 -> DataSource_SADA/1
  In1/1 -> Demux/1
  Demux/1 -> Cmd_Moror/1
  Demux/2 -> SadaStep_FC/1
  Demux/3 -> QvAgl_FC/1
  Demux/5 -> DataSource_QV/1

== system GS_model/Subsystem2/EquipmentCmd/Motor1 ==
  note: AA真采集
      | 55伪采集
  SADAQV_Cmd_Test : Inport
  Cmd_Motor : Inport  Port=2
  SadaStep_FC : Inport  Port=3
  QVAgl_FC : Inport  Port=4
  DataSource_SADA : Inport  Port=5
  DataSource_QV : Inport  Port=6
  Constant2 : Constant  Value=TestMode
  Data Store Memory : DataStoreMemory  DataStoreName=SadaAgl_FC  ReadBeforeWriteMsg=warning  WriteAfterWriteMsg=warning  WriteAfterReadMsg=warning  InitialValue=[0;0;0;0;0;0]  ShowAdditionalParam=off
  Data Store Memory4 : DataStoreMemory  DataStoreName=QvAgl_FC  ReadBeforeWriteMsg=warning  WriteAfterWriteMsg=warning  WriteAfterReadMsg=warning  InitialValue=[0;0;0;0]  ShowAdditionalParam=off
  Data Store Read2 : DataStoreRead  DataStoreName=SadaAgl_FC
  Data Store Read3 : DataStoreRead  DataStoreName=QvAgl_FC
  Data Store Write2 : DataStoreWrite  DataStoreName=QvAgl_FC
  Data Store Write3 : DataStoreWrite  DataStoreName=SadaAgl_FC
  Gain : Gain  Gain=180/pi
  Gain1 : Gain  Gain=180/pi
  Mux : Mux  Inputs=3
  Switch : Switch  Criteria=u2 > Threshold  Threshold=0.5
  Terminator : Terminator
  Terminator1 : Terminator
  Cmd_Moror : Outport
  wires:
  Constant2/1 -> Switch/2
  SADAQV_Cmd_Test/1 -> Switch/1
  Cmd_Motor/1 -> Switch/3  "20"
  QVAgl_FC/1 -> Gain1/1
  DataSource_SADA/1 -> Terminator/1
  DataSource_QV/1 -> Terminator1/1
  SadaStep_FC/1 -> Gain/1
  Gain/1 -> Data Store Write3/1  "6"
  Gain1/1 -> Data Store Write2/1  "4"
  Switch/1 -> Mux/1
  Data Store Read2/1 -> Mux/2  "6"
  Mux/1 -> Cmd_Moror/1  "30"
  Data Store Read3/1 -> Mux/3  "4"

== system GS_model/Subsystem2/EquipmentCmd/Mt ==
  In1 : Inport
  Demux : Demux  Outputs=3
  Cmd_Mt_UDP : Outport
  Cmd_Mt_FC : Outport  Port=2
  Cmd_Mt_DataSour : Outport  Port=3
  wires:
  Demux/1 -> Cmd_Mt_UDP/1
  Demux/2 -> Cmd_Mt_FC/1
  Demux/3 -> Cmd_Mt_DataSour/1
  In1/1 -> Demux/1

== system GS_model/Subsystem2/EquipmentCmd/Mt1 ==
  M_Cmd_Test : Inport
  UDP : Inport  Port=2
  FC : Inport  Port=3
  DataSource : Inport  Port=4
  Cmd_Mt_Analysis : Subsystem
  Constant4 : Constant  Value=TestMode
  Data Store Memory1 : DataStoreMemory  DataStoreName=Dyn_MtCmd_UDP  ReadBeforeWriteMsg=warning  WriteAfterWriteMsg=warning  WriteAfterReadMsg=warning  InitialValue=zeros(12,1)  ShowAdditionalParam=off
  Data Store Memory2 : DataStoreMemory  DataStoreName=Dyn_MtCmd_FC  ReadBeforeWriteMsg=warning  WriteAfterWriteMsg=warning  WriteAfterReadMsg=warning  InitialValue=zeros(12,1)  ShowAdditionalParam=off
  Data Store Memory3 : DataStoreMemory  DataStoreName=Dyn_MtCmd_Source  ReadBeforeWriteMsg=warning  WriteAfterWriteMsg=warning  WriteAfterReadMsg=warning  InitialValue=hex2dec('55')  ShowAdditionalParam=off
  Data Store Read1 : DataStoreRead  DataStoreName=Dyn_MtCmd_UDP
  Data Store Read2 : DataStoreRead  DataStoreName=Dyn_MtCmd_FC
  Data Store Read3 : DataStoreRead  DataStoreName=Dyn_MtCmd_Source
  Data Store Write1 : DataStoreWrite  DataStoreName=Dyn_MtCmd_UDP
  Data Store Write2 : DataStoreWrite  DataStoreName=Dyn_MtCmd_FC
  Data Store Write3 : DataStoreWrite  DataStoreName=Dyn_MtCmd_Source
  Switch1 : Switch  Criteria=u2 > Threshold  Threshold=0.5
  Cmd_Mt : Outport
  wires:
  Data Store Read1/1 -> Cmd_Mt_Analysis/1(udp_Mt)
  Data Store Read2/1 -> Cmd_Mt_Analysis/2(FC_Mt)
  Data Store Read3/1 -> Cmd_Mt_Analysis/3(Mt_Data_Source)
  UDP/1 -> Data Store Write1/1
  FC/1 -> Data Store Write2/1
  DataSource/1 -> Data Store Write3/1
  M_Cmd_Test/1 -> Switch1/1
  Cmd_Mt_Analysis/1(Cmd_Mt_Pro) -> Switch1/3
  Constant4/1 -> Switch1/2
  Switch1/1 -> Cmd_Mt/1

== system GS_model/Subsystem2/EquipmentCmd/PanelSpread ==
  In1 : Inport
  double→8lowbit : Subsystem
  Cmd_Spread : Outport
  wires:
  In1/1 -> double→8lowbit/1(In1)
  double→8lowbit/1(Out1) -> Cmd_Spread/1

== system GS_model/Subsystem2/Subsystem/Actuator ==
  Tc_Mt : Inport
  Tc_SADA : Inport  Port=2
  Tc_QV : Inport  Port=3
  Tc_Engine : Inport  Port=4
  Tc_Fw : Inport  Port=5
  Tc_Reset : Inport  Port=6
  UTC_1970 : Inport  Port=7
  Cmd_Fw : Inport  Port=8
  Cmd_Mt : Inport  Port=9
  Cmd_Motor : Inport  Port=10
  Cmd_Engine : Inport  Port=11
  Engine : Subsystem
      mask Display: disp('EngineModel')
  FlyWheel : Subsystem
      mask Display: disp('FWModel')
  Magnetorquer : Subsystem
      mask Display: disp('MtModel')
  Motor : Subsystem
      mask Display: disp('MotorModel')
  Selector3 : Selector  InputPortWidth=2  IndexOptions=Index vector (dialog)  Indices=2  OutputSizes=1
  Data_Fw : Outport
  Data_Mt : Outport  Port=2
  Data_SADA : Outport  Port=3
  Data_QV : Outport  Port=4
  T_Engine : Outport  Port=5
  F_Engine : Outport  Port=6
  M_Mt : Outport  Port=7
  Fw_H : Outport  Port=8
  Fw_T : Outport  Port=9
  Motor_Agl/w/a : Outport  Port=10
  wires:
  Tc_SADA/1 -> Motor/3(Tc_SADA)
  Cmd_Motor/1 -> Motor/2(Cmd_Motor)
  Tc_QV/1 -> Motor/4(Tc_QV)
  Cmd_Mt/1 -> Magnetorquer/2(Cmd_Mt)
  Cmd_Fw/1 -> FlyWheel/2(Cmd_FW)
  Tc_Engine/1 -> Engine/1(Tc_F_Engine)
  Cmd_Engine/1 -> Engine/2(Cmd_Engine)
  Magnetorquer/1(Data_Mt) -> Data_Mt/1
  Motor/2(Data_SADA) -> Data_SADA/1
  FlyWheel/1(Data_FW) -> Data_Fw/1
  Tc_Mt/1 -> Magnetorquer/1(Tc_Mt)
  Magnetorquer/2(M_Mt) -> M_Mt/1
  Tc_Fw/1 -> FlyWheel/3(TC_FW)
  Tc_Reset/1 -> Selector3/1
  FlyWheel/2(FW_Tw) -> Fw_T/1
  FlyWheel/3(FW_Hw) -> Fw_H/1
  Motor/3(Data_QV) -> Data_QV/1
  [Cent] -> Engine/3(Cent)
  Engine/1(T_Engine) -> T_Engine/1
  Engine/2(F_EP) -> F_Engine/1
  Motor/1(Motor_Agl/w/a) -> Motor_Agl/w/a/1
  Selector3/1 -> Motor/1(Att_Reset), FlyWheel/1(AttReset)
  UTC_1970/1 -> Motor/5(UTC_1970)

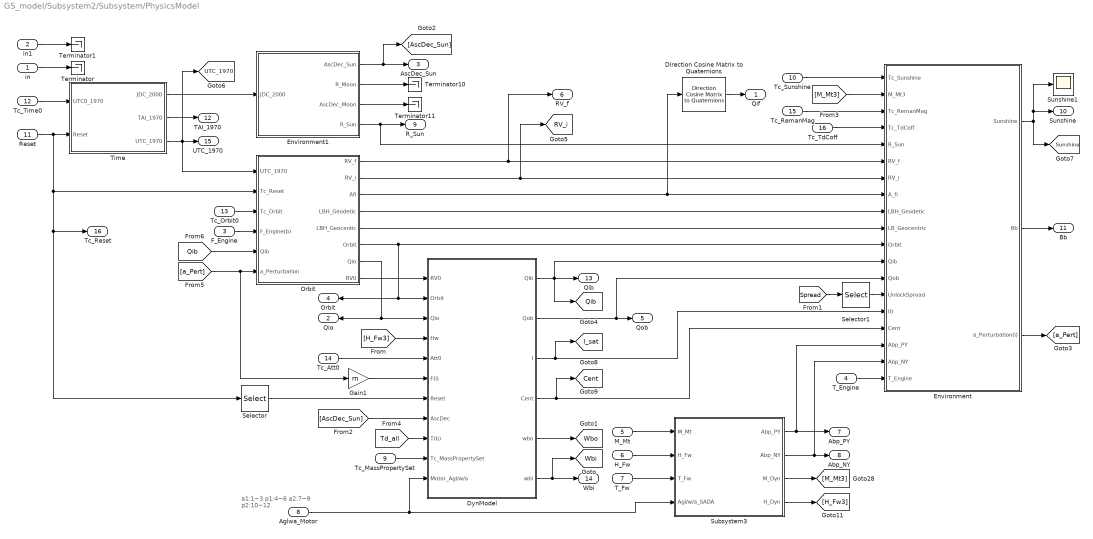
== system GS_model/Subsystem2/Subsystem/PhysicsModel ==
  note: a1:1~3
      | p1:4~6
      | a2:7~9
      | p2:10~12
  in : Inport
  in1 : Inport  Port=2
  F_Engine : Inport  Port=3
  T_Engine : Inport  Port=4
  M_Mt : Inport  Port=5
  H_Fw : Inport  Port=6
  T_Fw : Inport  Port=7
  Aglwa_Motor : Inport  Port=8
  Tc_MassPropertySet : Inport  Port=9
  Tc_Sunshine : Inport  Port=10
  Reset : Inport  Port=11
  Tc_Time0 : Inport  Port=12
  Tc_Orbit0 : Inport  Port=13
  Tc_Att0 : Inport  Port=14
  Tc_RemanMag : Inport  Port=15
  Tc_TdCoff : Inport  Port=16
  Direction Cosine Matrix to Quaternions : sharedtransform/Direction Cosine Matrix  to Quaternions  aMode=0  action=None  tolerance=eps(2)
      settings: SourceProductBaseCode=AE,PW,MT,VE,VP
  DynModel : Subsystem
      mask Display: disp('Attitude')
  Environment : Subsystem
      mask Display: disp('Environment')
  Environment1 : Subsystem
      mask Display: disp(['Sun','\n','Moon'])
  Gain1 : Gain  Gain=m
  Orbit : Subsystem
      mask Display: disp('Orbit')
  Selector : Selector  InputPortWidth=2  IndexOptions=Index vector (dialog)  Indices=2  OutputSizes=1
  Selector1 : Selector  InputPortWidth=8  IndexOptions=Index vector (dialog)  Indices=[1 2]  OutputSizes=1
  Subsystem3 : Subsystem
  Sunshine1 : Scope
  Terminator{,1,10..11} (4 alike) : Terminator
  Time : Subsystem
      mask Display: disp('Time')
  Qif : Outport
  Qio : Outport  Port=2
  AscDec_Sun : Outport  Port=3
  "Orbit " : Outport  Port=4
  Qob : Outport  Port=5
  RV_f : Outport  Port=6
  Abp_PY : Outport  Port=7
  Abp_NY : Outport  Port=8
  R_Sun : Outport  Port=9
  Sunshine : Outport  Port=10
  Bb : Outport  Port=11
  TAI_1970 : Outport  Port=12
  Qib : Outport  Port=13
  Wbi : Outport  Port=14
  UTC_1970 : Outport  Port=15
  Tc_Reset : Outport  Port=16
  tag scope: Cent=global, I_sat=global, Qib=global, RV_i=global, Sunshine=global, UTC_1970=global, Wbi=global, Wbo=global
  wires:
  [M_Mt3] -> Environment/2(M_Mt3)
  Orbit/7(Qio) -> Qio/1, DynModel/3(Qio)
  DynModel/1(Qib) -> Environment/12(Qib), [Qib], Qib/1
  Tc_Orbit0/1 -> Orbit/3(Tc_Orbit)
  Environment/2(Bb) -> Bb/1
  DynModel/2(Qob) -> Environment/13(Qob), Qob/1
  Environment1/1(AscDec_Sun) -> AscDec_Sun/1, [AscDec_Sun]
  Environment/1(Sunshine) -> Sunshine1/1, Sunshine/1, [Sunshine]
  DynModel/6(wbi) -> Wbi/1, [Wbi]
  Reset/1 -> Time/2(Reset), Tc_Reset/1, Selector/1, Orbit/2(Tc_Reset)
  Orbit/6(Orbit) -> Environment/11(Orbit), "Orbit "/1, DynModel/2(Orbit)
  Time/2(TAI_1970) -> TAI_1970/1
  Environment1/3(AscDec_Moon) -> Terminator11/1
  Environment1/2(R_Moon) -> Terminator10/1
  Orbit/3(Afi) -> Direction Cosine Matrix to Quaternions/1, Environment/8(A_fi)
  DynModel/5(wbo) -> [Wbo]
  Time/1(JDC_2000) -> Environment1/1(JDC_2000)
  Orbit/1(RV_f) -> Environment/6(RV_f), RV_f/1
  Tc_Time0/1 -> Time/1(UTC0_1970)
  Subsystem3/2(Abp_NY) -> Environment/18(Abp_NY), Abp_NY/1
  Subsystem3/1(Abp_PY) -> Environment/17(Abp_PY), Abp_PY/1
  Time/3(UTC_1970) -> Orbit/1(UTC_1970), [UTC_1970], UTC_1970/1
  Tc_RemanMag/1 -> Environment/3(Tc_RemanMag)
  Orbit/2(RV_i) -> Environment/7(RV_i), [RV_i]
  Tc_TdCoff/1 -> Environment/4(Tc_TdCoff)
  [a_Pert] -> Gain1/1, Orbit/6(a_Perturbation)
  Environment/3(a_Perturbation(i)) -> [a_Pert]
  Orbit/4(LBH_Geodetic) -> Environment/9(LBH_Geodetic)
  Orbit/5(LBH_Geocentic) -> Environment/10(LB_Geocentric)
  Environment1/4(R_Sun) -> Environment/5(R_Sun), R_Sun/1
  [Spread] -> Selector1/1
  Orbit/8(RV0) -> DynModel/1(RV0)
  Tc_Att0/1 -> DynModel/5(Att0)
  Gain1/1 -> DynModel/6(F(i))
  [AscDec_Sun] -> DynModel/8(AscDec)
  Selector/1 -> DynModel/7(Reset)
  [H_Fw3] -> DynModel/4(Hw)
  Subsystem3/3(M_Dyn) -> [M_Mt3]
  Subsystem3/4(H_Dyn) -> [H_Fw3]
  Aglwa_Motor/1 -> Subsystem3/4(Agl/w/a_SADA), DynModel/11(Motor_Agl/w/a)
  M_Mt/1 -> Subsystem3/1(M_Mt)
  H_Fw/1 -> Subsystem3/2(H_Fw)
  T_Fw/1 -> Subsystem3/3(T_Fw)
  [Td_all] -> DynModel/9(T(b))
  Tc_Sunshine/1 -> Environment/1(Tc_Sunshine)
  Tc_MassPropertySet/1 -> DynModel/10(Tc_MassPropertySet)
  DynModel/3(I) -> Environment/15(I0), [I_sat]
  DynModel/4(Cent) -> Environment/16(Cent), [Cent]
  [Qib] -> Orbit/5(Qib)
  F_Engine/1 -> Orbit/4(F_Engine(b))
  Selector1/1 -> Environment/14(UnlockSpread)
  Direction Cosine Matrix to Quaternions/1 -> Qif/1
  in/1 -> Terminator/1
  in1/1 -> Terminator1/1
  T_Engine/1 -> Environment/19(T_Engine)

== system GS_model/Subsystem2/Subsystem/Sensor ==
  M_Mt : Inport
  Qob : Inport  Port=2
  RV_f : Inport  Port=3
  Abp_PY : Inport  Port=4
  Abp_NY : Inport  Port=5
  R_Sun(i) : Inport  Port=6
  Sunshine : Inport  Port=7
  Bb : Inport  Port=8
  TAI_1970 : Inport  Port=9
  Qib : Inport  Port=10
  Wbi_b : Inport  Port=11
  UTC_1970 : Inport  Port=12
  Tc_Reset : Inport  Port=13
  Tc_St : Inport  Port=14
  Tc_Gyro : Inport  Port=15
  Tc_Ass : Inport  Port=16
  Tc_Mm : Inport  Port=17
  Tc_GNSS : Inport  Port=18
  Ass : Subsystem
      mask Display: disp('Ass(Body&Panel)\nModel')
  GNSS : Subsystem
      mask Display: disp('GNSS')
  Gyro : Subsystem
      mask Display: disp('GyroModel')
  Magnetometer : Subsystem
      mask Display: disp('MagA&B&C&D\nModel')
  MatrixMultiply : Product  Multiplication=Matrix(*)
  Normalize Vector : vrlib/Utilities/Normalize Vector  maxzero=0
  Quaternions to Direction Cosine Matrix : sharedtransform/Quaternions to  Direction Cosine Matrix  aMode=aMode
      settings: SourceProductBaseCode=AE,PW,MT,VE,VP
  StA&B&C&DModel1 : Subsystem
      mask Display: disp('StA&B&C&D\nModel')
  Sun_b : Scope
  TC_Reset : Outport
  RV_f_out : Outport  Port=2
  Qob_out : Outport  Port=3
  Data_St : Outport  Port=4
  Data_Gyro : Outport  Port=5
  Data_Ass : Outport  Port=6
  Data_Mm : Outport  Port=7
  Data_GNSS : Outport  Port=8
  tag scope: Sun_b=global
  wires:
  Qib/1 -> Quaternions to Direction Cosine Matrix/1, StA&B&C&DModel1/1(Qib)
  Tc_St/1 -> StA&B&C&DModel1/4(TC_St)
  Tc_Gyro/1 -> Gyro/2(Tc_Gyro)
  Wbi_b/1 -> Gyro/1(Wbi_b)
  Bb/1 -> Magnetometer/1(Bb)
  Tc_Mm/1 -> Magnetometer/3(Tc_Mm)
  Gyro/1(Data_Gyro) -> Data_Gyro/1
  Tc_GNSS/1 -> GNSS/2(TC_GNSS)
  RV_f/1 -> GNSS/1(RV_f), RV_f_out/1
  Magnetometer/1(Data_Mm) -> Data_Mm/1
  GNSS/1(Data_GNSS) -> Data_GNSS/1
  UTC_1970/1 -> GNSS/4(UTC_1970), StA&B&C&DModel1/5(UTC_1970)
  StA&B&C&DModel1/1(TM_St) -> Data_St/1
  Quaternions to Direction Cosine Matrix/1 -> MatrixMultiply/1
  Tc_Ass/1 -> Ass/3(TC_Ass)
  Abp_PY/1 -> Ass/4(Abp_PY)
  Abp_NY/1 -> Ass/5(Abp_NY)
  MatrixMultiply/1 -> Sun_b/1, StA&B&C&DModel1/2(Sun_b), Ass/1(Sun_b), [Sun_b]
  Ass/1(Data_Ass) -> Data_Ass/1
  R_Sun(i)/1 -> Normalize Vector/1
  TAI_1970/1 -> GNSS/3(TAI1970)
  M_Mt/1 -> Magnetometer/2(M_Mt)
  Normalize Vector/1 -> MatrixMultiply/2
  Sunshine/1 -> Ass/2(Sunshine), StA&B&C&DModel1/3(Sunshine)
  Qob/1 -> Qob_out/1, StA&B&C&DModel1/6(Qob)
  Tc_Reset/1 -> TC_Reset/1

== system GS_model/Subsystem2/Tc/Ass1 ==
  note: Dyn_AssCurGNDSet_Choice
      | Dyn_AssCurGNDSet_Switch
      | Dyn_AssCurGNDSet_A1
      | Dyn_AssCurGNDSet_A2
      | Dyn_AssCurGNDSet_A3
      | Dyn_AssCurGNDSet_A4
      | Dyn_AssErr_Constant_Choice
      | Dyn_AssErr_Constant_Switch
      | Dyn_AssErr_WildValue_Choice
      | Dyn_AssErr_WildValue_Switch
      | Dyn_AssErr_Jump_Choice
      | Dyn_AssErr_Jump_Switch
      | Dyn_AssErr_Jump_TSet
      | Dyn_AssErr_Jump_AmpCoffSet
      | Dyn_AssErr_Wave_Choice
      | Dyn_AssErr_Wave_Switch
      | Dyn_AssErr_Wave_AmpCoffSet
  In1 : Inport
  Constant : Constant  Value=zeros(17,1)
  Constant2 : Constant  Value=TestMode
  Data Store Memory10 : DataStoreMemory  DataStoreName=Dyn_AssErr_Jump  ReadBeforeWriteMsg=warning  WriteAfterWriteMsg=warning  WriteAfterReadMsg=warning  InitialValue=[0;0;0;0]  ShowAdditionalParam=off
  Data Store Memory14 : DataStoreMemory  DataStoreName=Dyn_AssErr_Wave  ReadBeforeWriteMsg=warning  WriteAfterWriteMsg=warning  WriteAfterReadMsg=warning  InitialValue=[0;0;0]  ShowAdditionalParam=off
  Data Store Memory17 : DataStoreMemory  DataStoreName=Dyn_AssErr_Constant  ReadBeforeWriteMsg=warning  WriteAfterWriteMsg=warning  WriteAfterReadMsg=warning  InitialValue=[1;0]  ShowAdditionalParam=off
  Data Store Memory4 : DataStoreMemory  DataStoreName=Dyn_AssCurGNDSet  ReadBeforeWriteMsg=warning  WriteAfterWriteMsg=warning  WriteAfterReadMsg=warning  InitialValue=[1;0;0;0;0;0]  ShowAdditionalParam=off
  Data Store Memory8 : DataStoreMemory  DataStoreName=Dyn_AssErr_WildValue  ReadBeforeWriteMsg=warning  WriteAfterWriteMsg=warning  WriteAfterReadMsg=warning  InitialValue=[0;0]  ShowAdditionalParam=off
  Data Store Read10 : DataStoreRead  DataStoreName=Dyn_AssErr_Jump
  Data Store Read14 : DataStoreRead  DataStoreName=Dyn_AssErr_Wave
  Data Store Read17 : DataStoreRead  DataStoreName=Dyn_AssErr_Constant
  Data Store Read4 : DataStoreRead  DataStoreName=Dyn_AssCurGNDSet
  Data Store Read8 : DataStoreRead  DataStoreName=Dyn_AssErr_WildValue
  Data Store Write10 : DataStoreWrite  DataStoreName=Dyn_AssErr_Jump
  Data Store Write14 : DataStoreWrite  DataStoreName=Dyn_AssErr_Wave
  Data Store Write17 : DataStoreWrite  DataStoreName=Dyn_AssErr_Constant
  Data Store Write4 : DataStoreWrite  DataStoreName=Dyn_AssCurGNDSet
  Data Store Write8 : DataStoreWrite  DataStoreName=Dyn_AssErr_WildValue
  Demux : Demux  Outputs=[6;2;2;4;3]
  Mux : Mux  Inputs=5
  Switch : Switch  Criteria=u2 > Threshold  Threshold=0.5
  Tc_Ass : Outport
  wires:
  Switch/1 -> Demux/1
  Constant/1 -> Switch/1
  Constant2/1 -> Switch/2
  Mux/1 -> Tc_Ass/1
  Demux/1 -> Data Store Write4/1
  Demux/2 -> Data Store Write17/1
  Demux/3 -> Data Store Write8/1
  Demux/4 -> Data Store Write10/1
  Demux/5 -> Data Store Write14/1
  Data Store Read8/1 -> Mux/3
  Data Store Read17/1 -> Mux/2
  Data Store Read10/1 -> Mux/4
  Data Store Read4/1 -> Mux/1
  Data Store Read14/1 -> Mux/5
  In1/1 -> Switch/3

== system GS_model/Subsystem2/Tc/Att1 ==
  Att0 : Inport
  in : Inport  Port=2
  Constant1 : Constant  Value=TestMode
  Data Store Memory : DataStoreMemory  DataStoreName=Att0  ReadBeforeWriteMsg=warning  WriteAfterWriteMsg=warning  WriteAfterReadMsg=warning  InitialValue=[Agl0;Wbi0]  ShowAdditionalParam=off
  Data Store Read : DataStoreRead  DataStoreName=Att0
  Data Store Write : DataStoreWrite  DataStoreName=Att0
  Gain : Gain  Gain=DEG2RAD
  Switch : Switch  Criteria=u2 > Threshold  Threshold=0.5
  Tc_Att0 : Outport
  wires:
  Data Store Read/1 -> Tc_Att0/1
  Att0/1 -> Switch/1
  Constant1/1 -> Switch/2
  Switch/1 -> Data Store Write/1
  Gain/1 -> Switch/3
  in/1 -> Gain/1

== system GS_model/Subsystem2/Tc/Engine1 ==
  note: Dyn_FireDir_Bias_Choice
      | Dyn_FireDir_Bias_Switch
      | Dyn_FireDir_Bias_X
      | Dyn_FireDir_Bias_Y
      | Dyn_FireDir_Bias_Z
      | Dyn_EngineFSet_Choice
      | Dyn_EngineFSet_Switch
      | Dyn_EngineFSet_FValue
      | Dyn_EngineFirePauseSet_Choice
      | Dyn_EngineFirePauseSet_Switch
      | Dyn_EngineFirePauseSet_Value
  in : Inport
  Constant : Constant  Value=zeros(11,1)
  Constant2 : Constant  Value=TestMode
  Data Store Memory : DataStoreMemory  DataStoreName=Dyn_EngineSet  ReadBeforeWriteMsg=warning  WriteAfterWriteMsg=warning  WriteAfterReadMsg=warning  InitialValue=zeros(11,1)  ShowAdditionalParam=off
  Data Store Read : DataStoreRead  DataStoreName=Dyn_EngineSet
  Data Store Write : DataStoreWrite  DataStoreName=Dyn_EngineSet
  Switch : Switch  Criteria=u2 > Threshold  Threshold=0.5
  Tc_Eg : Outport
  wires:
  in/1 -> Switch/3
  Data Store Read/1 -> Tc_Eg/1
  Constant/1 -> Switch/1
  Switch/1 -> Data Store Write/1
  Constant2/1 -> Switch/2
